simulink model "TriggerEdge2_2018a"  (R2018a)
settings: Solver=FixedStepAuto  StartTime=0.0  StopTime=10.0  FixedStep=0.1  MaxStep=1  RelTol=1e-3
settings Model: Creator=86188  LastModifiedBy=bzhan

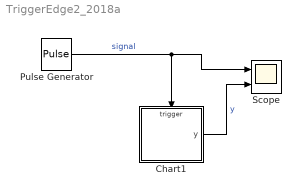
== system TriggerEdge2_2018a ==
  Chart1 : Stateflow chart  TreatAsAtomicUnit=on
  Pulse Generator : DiscretePulseGenerator  PulseType=Time based  Period=1  PulseWidth=50
  Scope : Scope  NumInputPorts=2
  wires:
  Pulse Generator/1 -> Scope/1, Chart1/Trigger  "signal"
  Chart1/1(y) -> Scope/2  "y"

== stateflow chart TriggerEdge2_2018a/Chart1 ==
  settings: executeAtInitialization=1
  state AA
    du: y = y + 1
  (default) -> AA
  data: y output =0
  events: out_cmd input FALLING_EDGE_EVENT
